simulink model "SdC_progetto"  (R2023b)
settings: Solver=VariableStepAuto  StartTime=0.0  StopTime=0.01  RelTol=1e-3
values from neighbouring files (symbols this model uses):
  C = [1 0]    [progetto.m]
  u_e = beta * omega_e + k * theta_e    (= 52.3598775598)    [progetto.m]
  W = w    [progetto.m]
  x_e = [theta_e; omega_e]    [progetto.m]
  x_sim = x_e    [progetto.m]
libraries: simulink x2, cstblocks x1
settings Model: Creator=guidocarnevale  LastModifiedBy=loren

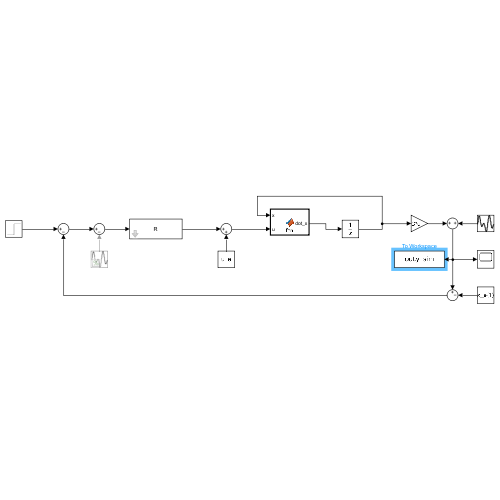
[thumbnail: Simulink's stored preview of the top-level diagram]
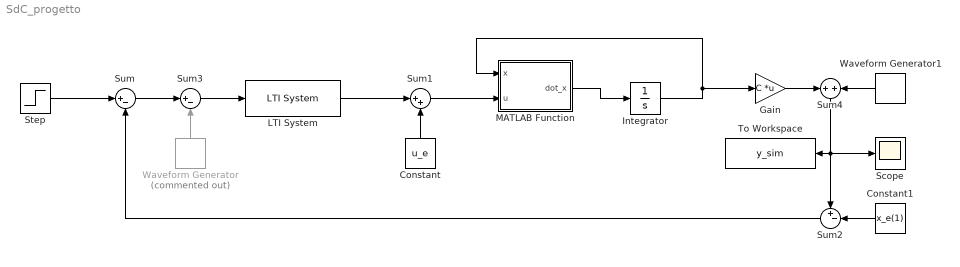
== system SdC_progetto ==
  Constant : Constant  Value=u_e
  Constant1 : Constant  Value=x_e(1)
  Gain : Gain  Gain=C  Multiplication=Matrix(K*u)
  Integrator : Integrator  InitialCondition=x_sim
  LTI System : cstblocks/LTI System  Tag=R  sys=R  IC=[]  PadeOrder=0
  MATLAB Function : MATLAB Function  TreatAsAtomicUnit=on
  Scope : Scope
  Step : Step  Time=0  After=W  SampleTime=0
  Sum : Sum  Inputs=|+-
  Sum1 : Sum  Inputs=|++
  Sum2 : Sum  Inputs=+-|
  Sum3 : Sum  Inputs=|+-
  Sum4 : Sum  Inputs=+|+
  To Workspace : ToWorkspace  VariableName=y_sim  SaveFormat=Timeseries  SampleTime=-1
  Waveform Generator : simulink/Sources/Waveform Generator  Commented=on  OutMin=[]  OutMax=[]  OutDataTypeStr=double  SelectedSignal=1  Signals=sin(1, 5e4, 0)+sin(1, 10e4, 0)+sin(1, 15e4, 0)+sin(1, 20e4, 0)  BlockNames=MultiportSwitch_3ff6c47c90af40d  SampleTime=0.0000001
  Waveform Generator1 : simulink/Sources/Waveform Generator  OutMin=[]  OutMax=[]  OutDataTypeStr=double  SelectedSignal=1  Signals=sin(1, 0.1, 0)+sin(1, 0.2, 0)+sin(1, 0.3, 0)+sin(1, 0.4, 0)  BlockNames=MultiportSwitch_f54722ed020749d  SampleTime=0.01
  wires:
  MATLAB Function/1(dot_x) -> Integrator/1
  Integrator/1 -> MATLAB Function/1(x), Gain/1
  Sum/1 -> Sum3/1
  LTI System/1 -> Sum1/1
  Constant/1 -> Sum1/2
  Sum1/1 -> MATLAB Function/2(u)
  Sum3/1 -> LTI System/1
  Waveform Generator1/1 -> Sum4/2
  Gain/1 -> Sum4/1
  Sum4/1 -> To Workspace/1, Scope/1, Sum2/1
  Constant1/1 -> Sum2/2
  Sum2/1 -> Sum/2
  Waveform Generator/1 -> Sum3/2
  Step/1 -> Sum/1

== matlab function SdC_progetto/MATLAB Function ==
  data: x input; u input; dot_x output
function dot_x = fcn(x,u)

J0 = 1.7;
Ji =    [1     0.7    0.09    0.02];
phi =   [-0.04   2.9     2.8     -2.6];
k = 50;
J = @(x) J0 + Ji(1) * cos(x + phi(1))+ Ji(2) * cos(2*x + phi(2))+ Ji(3) * cos(3*x + phi(3))+ Ji(4) * cos(4*x + phi(4));
beta=1;

dot_x = zeros(2,1);

dot_x(1) = x(2);

dot_x(2) = u/J(x(1)) - (beta*x(2))/J(x(1)) - (k*x(1))/J(x(1));
